simulink model "sim_devel"  (R2025b)
settings: Solver=VariableStepAuto  StartTime=0.0  StopTime=40  RelTol=1e-3
InitFcn:
  | simstruct_init(0);
libraries: devel_lib x1
settings Model: PacingRate=3  Creator=nicolls  LastModifiedBy=nicolls

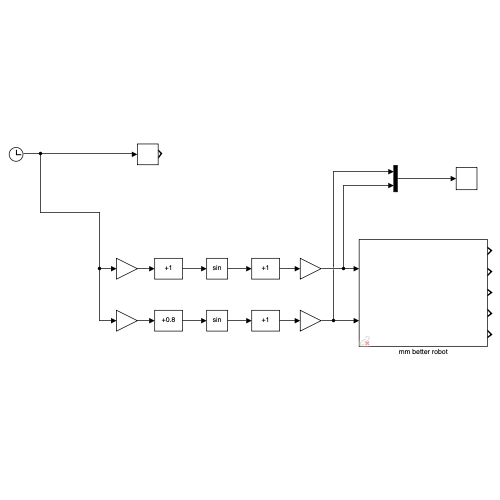
[thumbnail: Simulink's stored preview of the top-level diagram]
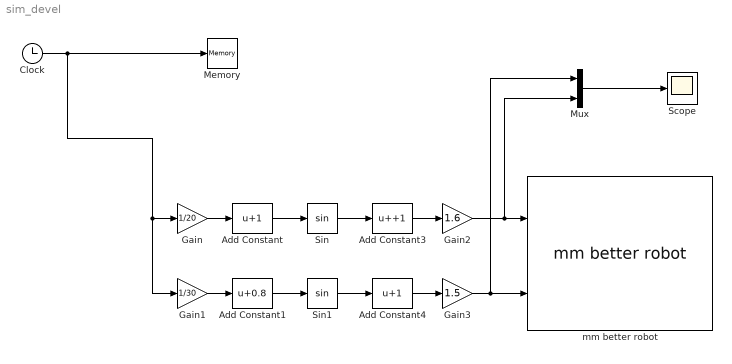
== system sim_devel ==
  Add Constant : Bias  Bias=1  SaturateOnIntegerOverflow=off
  Add Constant1 : Bias  Bias=0.8  SaturateOnIntegerOverflow=off
  Add Constant3 : Bias  Bias=+1  SaturateOnIntegerOverflow=off
  Add Constant4 : Bias  Bias=1  SaturateOnIntegerOverflow=off
  Clock : Clock
  Gain : Gain  Gain=1/20
  Gain1 : Gain  Gain=1/30
  Gain2 : Gain  Gain=1.6
  Gain3 : Gain  Gain=1.5
  Memory : Memory
  Mux : Mux  Inputs=2
  Scope : Scope
      settings: ActiveDisplayYMinimum=-1  ActiveDisplayYMaximum=1
  Sin : Trigonometry
  Sin1 : Trigonometry
  mm better robot : devel_lib/mm better robot  simstruct=simstruct
  wires:
  Clock/1 -> Gain1/1, Gain/1, Memory/1
  Gain/1 -> Add Constant/1
  Add Constant/1 -> Sin/1
  Gain1/1 -> Add Constant1/1
  Add Constant1/1 -> Sin1/1
  Sin/1 -> Add Constant3/1
  Gain2/1 -> mm better robot/1, Mux/2
  Sin1/1 -> Add Constant4/1
  Gain3/1 -> Mux/1, mm better robot/2
  Mux/1 -> Scope/1
  Add Constant3/1 -> Gain2/1
  Add Constant4/1 -> Gain3/1
